simulink model "Stinger"  (R2023a)
settings: Solver=VariableStepAuto  StartTime=0.0  StopTime=20  FixedStep=1e-3  EnableMultiTasking=on
values from neighbouring files (symbols this model uses):
  bp = 0.001    [ControlLawsScript.m]    (also in ControlLaws_Script.m)
  bq = 0.001    [ControlLawsScript.m]    (also in ControlLaws_Script.m)
  br = 0.001    [ControlLawsScript.m]    (also in ControlLaws_Script.m)
  cx = 5    [ControlLawsScript.m]    (also in ControlLaws_Script.m)
  cy = 5    [ControlLawsScript.m]    (also in ControlLaws_Script.m)
  cz = 5    [ControlLawsScript.m]    (also in ControlLaws_Script.m)
  g = 9.80665    [ControlLawsScript.m]    (also in ControlLaws_Script.m; Qball_X8_Model.m = 9.87)
  Kp = (Jx/Tc)-bp    (= 1.02772632451)    [ControlLawsScript.m]    (also in ControlLaws_Script.m = 4.11390529802)
  Kp2 = Jx*((4/ts))*((-4/ts)+((bp+Kp)/Jx))/Kp    (= 1.68163467643)    [ControlLawsScript.m]    (also in ControlLaws_Script.m = 6.72163348437)
  Kq = (Jy/Tc)-bq    (= 1.02971502036)    [ControlLawsScript.m]    (also in ControlLaws_Script.m = 4.12186008142)
  Kq2 = Jy*((4/ts))*((-4/ts)+((bq+Kq)/Jy))/Kq    (= 1.68163151937)    [ControlLawsScript.m]    (also in ControlLaws_Script.m = 6.72163033191)
  Kr = (Jz/Tc)-br    (= 1.98490876719)    [ControlLawsScript.m]    (also in ControlLaws_Script.m = 7.94263506876)
  Kr2 = Jz*((4/ts))*((-4/ts)+((br+Kr)/Jz))/Kr    (= 1.68084638651)    [ControlLawsScript.m]    (also in ControlLaws_Script.m = 6.72084606682)
  kv = 1/930    (= 0.0010752688172)    [StingerScript.m]
  Kx = abs(Kx)    [ControlLawsScript.m]    (also in ControlLaws_Script.m)
  Ky = abs(Ky)    [ControlLawsScript.m]    (also in ControlLaws_Script.m)
  Kz = (m/Tcz)-cz    (= 38.5143536865)    [ControlLawsScript.m]    (also in ControlLaws_Script.m)
  Kz2 = m*((4/tsz))*((-4/tsz)+((cz+Kz)/m))/Kz    (= 1.89810050529)    [ControlLawsScript.m]    (also in ControlLaws_Script.m)
  m = 3.4811482949175    (= 3.48114829492)    [ControlLawsScript.m]    (also in ControlLaws_Script.m; Qball_X8_Model.m = 1.45)
  pitch_angle_limit = pi/6    (= 0.523598775598)    [ControlLawsScript.m]    (also in ControlLaws_Script.m = 0.558505360638)
  R2D = 180/pi    (= 57.2957795131)    [ControlLawsScript.m]    (also in ControlLaws_Script.m)
  roll_angle_limit = pi/6    (= 0.523598775598)    [ControlLawsScript.m]    (also in ControlLaws_Script.m = 0.558505360638)
  z_x = cx    (= 5)    [ControlLawsScript.m]    (also in ControlLaws_Script.m)
  z_y = cy    (= 5)    [ControlLawsScript.m]    (also in ControlLaws_Script.m)
undefined symbols (not defined in the file or in its folder): FC, LAC, LeftAftArm, LeftAftProp, LeftAftSkid, LeftArm, LeftFrontArm, LeftFrontProp, LeftFrontSkid, LeftProp, Lower, missionPlanX, missionPlanY, missionPlanYaw, missionPlanZ, RAC, RightAftArm, RightAftProp, RightAftSkid, RightArm, RightFrontArm, RightFrontProp, RightFrontSkid, RightProp, SC, timeConstant, Upper, X, Y, Z
libraries: sm_lib x98, nesl_utility x56, fl_lib x45, ee_lib x19, batteryecm_lib x2, sharedtransformsys x1, sharedutil x1
(part 3 of 4)

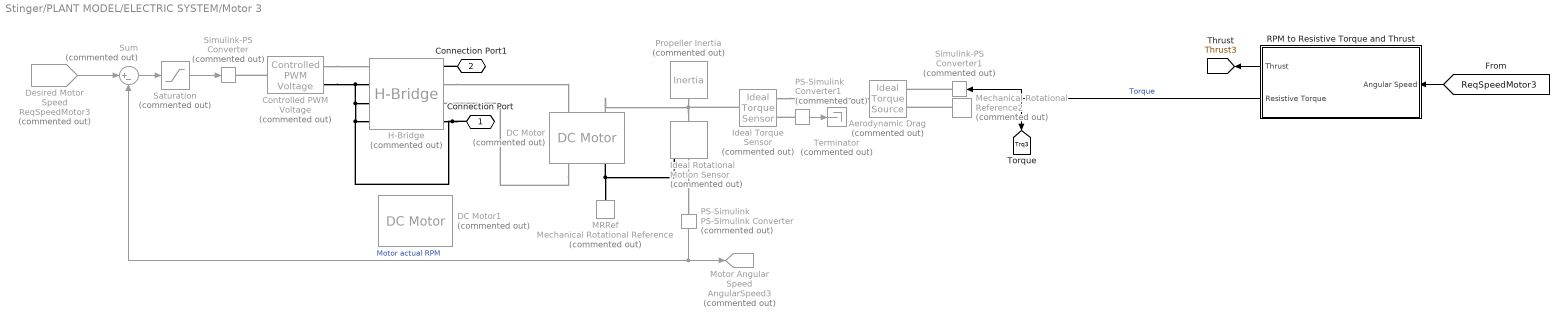
== system Stinger/PLANT MODEL/ELECTRIC SYSTEM/Motor 3 ==
  Aerodynamic Drag : fl_lib/Mechanical/Mechanical Sources/Ideal Torque Source  Commented=on
  Controlled PWM Voltage : ee_lib/Integrated Circuits/Controlled PWM Voltage  Commented=on  F=200 Hz  TD=0 s  pulse_width_offset=0 s  pulse_min=0 s  pwm_or_av=1  event_type=1  sample_time=5e-6 s  Vmin=0 V  Vmax=5 V  Vm=1 V  u_min=0  u_max=1
      settings: InternalSimscapePortConfiguration="{\"Bottom\":[],\"Left\":[{\"id\":\"u\",\"label\":\"u\",\"type\":\"input\"}],\"Right\":[{\"id\":\"p2\",\"label\":\"PWM\",\"type\":\"foundation.electrical.electrical\"},{\"id\":\"n2\",\"label\":\"REF\",\"type\":\"foundation.electrical.electrical\"}],\"Top\":[]}"
  DC Motor : ee_lib/Electromechanical/Brushed Motors/DC Motor  Commented=on  field_option=ee.enum.field_option.pm  Rf=100 Ohm  Lf=1 H  Laf=0.15 H  If0=0 A  parameterization=ee.enum.dcparam_option.circuit_param  Ra=R Ohm  La=100 uH  emf_or_torque=ee.enum.emf_or_torque.kv  Kv=kv V/rpm  Ki=kv N*m/A  T_stall=0.1 N*m  w_max=4000 rpm  w_rated=2500 rpm  P_rated=10 W  V_rated=12 V  lam_param=ee.enum.lam_param.current  i_noload=Ic A  V_i_noload=14.8 V  J=0 kg*m^2  lam=0.5e-5 N*m/(rad/s)  speed0=0 rpm  enable_fault_armature=simscape.enum.onoff.off  rev_faulted=1 / 3  G_faulted_armature=1e-5 S  fault_trigger_armature=ee.enum.faults.faultTrigger.temporal  t_fault_armature=1 s  max_permissible_current_armature=inf A  t_fail_on_current_armature=1 s  enable_fault_field=simscape.enum.onoff.off  G_faulted_field=1e-5 S  fault_trigger_field=ee.enum.faults.faultTrigger.temporal  t_fault_field=1 s  max_permissible_current_field=inf A  t_fail_on_current_field=1 s  fault_action=simscape.enum.assert.action.none  alpha=3.93e-3 1/K  Tmeas=25 degC  thermal_mass=100 J/K  initial_temperature=25 degC
  DC Motor1 : ee_lib/Electromechanical/Brushed Motors/DC Motor  Commented=on  field_option=ee.enum.field_option.pm  Rf=100 Ohm  Lf=1 H  Laf=0.15 H  If0=0 A  parameterization=ee.enum.dcparam_option.circuit_param  Ra=R Ohm  La=100 uH  emf_or_torque=ee.enum.emf_or_torque.kv  Kv=kv V/rpm  Ki=kv N*m/A  T_stall=0.1 N*m  w_max=4000 rpm  w_rated=2500 rpm  P_rated=10 W  V_rated=12 V  lam_param=ee.enum.lam_param.current  i_noload=Ic A  V_i_noload=14.8 V  J=0 kg*m^2  lam=0.5e-5 N*m/(rad/s)  speed0=0 rpm  enable_fault_armature=simscape.enum.onoff.off  rev_faulted=1 / 3  G_faulted_armature=1e-5 S  fault_trigger_armature=ee.enum.faults.faultTrigger.temporal  t_fault_armature=1 s  max_permissible_current_armature=inf A  t_fail_on_current_armature=1 s  enable_fault_field=simscape.enum.onoff.off  G_faulted_field=1e-5 S  fault_trigger_field=ee.enum.faults.faultTrigger.temporal  t_fault_field=1 s  max_permissible_current_field=inf A  t_fail_on_current_field=1 s  fault_action=simscape.enum.assert.action.none  alpha=3.93e-3 1/K  Tmeas=25 degC  thermal_mass=100 J/K  initial_temperature=25 degC
  Desired Motor Speed : From  Commented=on  GotoTag=ReqSpeedMotor3  TagVisibility=global
  H-Bridge : ee_lib/Semiconductors & Converters/Converters/H-Bridge  Commented=on  supply_ports=ee.enum.supply_ports.showsupply  pwm_or_av=ee.enum.pwm_or_av.pwm  regenerative_braking_mode=ee.enum.converters.regenerative_braking_mode.always_enabled  discontinuous=ee.enum.current_profile.continuous  freewheeling_mode=ee.enum.converters.freewheeling_mode.two_switches_one_diode  Rload=3.38+0.1 Ohm  Lload=1e-5 H  F=4 kHz  Venable=0.01 V  Vmax=5 V  Vreverse=10000 V  Vbrake=10000 V  Vm=12 V  Ron=0.00001 Ohm  Don=0.1 Ohm  Goff=1e-6 S  Tmeas=298.15 K  Ron2=0.1 Ohm  Don2=0.05 Ohm  Tmeas2=398.15 K  thermal_mass=100 J/K  initial_temperature=298.15 K
      settings: InternalSimscapePortConfiguration="{\"Bottom\":[],\"Left\":[{\"id\":\"ENA\",\"label\":\"PWM\",\"type\":\"foundation.electrical.electrical\"},{\"id\":\"REF\",\"label\":\"REF\",\"type\":\"foundation.electrical.electrical\"},{\"id\":\"REV\",\"label\":\"REV\",\"type\":\"foundation.electrical.electrical\"},{\"id\":\"BRK\",\"label\":\"BRK\",\"type\":\"foundation.electrical.electrical\"}],\"Right\":[{\"id\":\"p1\",\"label\":\"V+\",\"type\":\"foundation.electrical.electrical\"},{\"id\":\"p2\",\"label\":\"+\",\"type\":\"foundation.electrical.electrical\"},{\"id\":\"n2\",\"label\":\"-\",\"type\":\"foundation.electrical.electrical\"},{\"id\":\"n1\",\"label\":\"V-\",\"type\":\"foundation.electrical.electrical\"}],\"Top\":[]}"
  Ideal Rotational Motion Sensor : fl_lib/Mechanical/Mechanical Sensors/Ideal Rotational Motion Sensor  Commented=on  reference=foundation.enum.MeasurementReference.difference  acceleration_port=false  velocity_port=true  position_port=true  wrap_angle=simscape.enum.onoff.off  offset=0 deg
  Ideal Torque Sensor : fl_lib/Mechanical/Mechanical Sensors/Ideal Torque Sensor  Commented=on
  MRRef : fl_lib/Mechanical/Rotational Elements/Mechanical Rotational Reference  Commented=on
  Mechanical Rotational Reference2 : fl_lib/Mechanical/Rotational Elements/Mechanical Rotational Reference  Commented=on
  Motor Angular Speed : Goto  Commented=on  GotoTag=AngularSpeed3  TagVisibility=global
  PS-Simulink : nesl_utility/PS-Simulink Converter  Commented=on  PhysicalDomain=network_engine_domain  SubClassName=ps_output  LeftPortType=input  RightPortType=output  PseudoPeriodic=off  Frequencies=[]  VectorFormat=1-D array  Unit=rpm  AffineConversion=off
  PS-Simulink Converter1 : nesl_utility/PS-Simulink Converter  Commented=on  PhysicalDomain=network_engine_domain  SubClassName=ps_output  LeftPortType=input  RightPortType=output  PseudoPeriodic=off  Frequencies=[]  VectorFormat=1-D array  Unit=inherit  AffineConversion=off
  Propeller Inertia : fl_lib/Mechanical/Rotational Elements/Inertia  Commented=on  inertia=J kg*m^2  num_ports=foundation.enum.numPorts2.one  w_specify=off  w_priority=High  w=0 rpm  w_nominal_specify=off  w_nominal_unit=rad/s  w_nominal_value=1  t_specify=off  t_priority=High  t=0 N*m  t_nominal_specify=off  t_nominal_unit=N*m  t_nominal_value=1
  RPM to Resistive Torque and Thrust : Subsystem
  Saturation : Saturate  Commented=on  UpperLimit=1  LowerLimit=0
  Simulink-PS Converter : nesl_utility/Simulink-PS Converter  Commented=on  PhysicalDomain=network_engine_domain  SubClassName=ps_input  LeftPortType=input  RightPortType=output  PseudoPeriodic=off  Frequencies=[]  NoiseDistribution=none  NoiseParameters=[]  Unit=1  AffineConversion=off  FilteringAndDerivatives=provide  SimscapeFilterOrder=1  InputFilterTimeConstant=0.001  UdotUserProvided=0
  Simulink-PS Converter1 : nesl_utility/Simulink-PS Converter  Commented=on  PhysicalDomain=network_engine_domain  SubClassName=ps_input  LeftPortType=input  RightPortType=output  PseudoPeriodic=off  Frequencies=[]  NoiseDistribution=none  NoiseParameters=[]  Unit=N*m  AffineConversion=off  FilteringAndDerivatives=provide  SimscapeFilterOrder=1  InputFilterTimeConstant=0.001  UdotUserProvided=0
  Sum : Sum  Commented=on  Inputs=|+-
  Terminator : Terminator  Commented=on
  Connection Port : PMIOPort  Side=Left
  Connection Port1 : PMIOPort  Port=2  Side=Right
  tag scope: Thrust3=global, Trq3=global
  wires:
  RPM to Resistive Torque and Thrust/2(Resistive Torque) -> Simulink-PS Converter1/1, [Trq3]  "Torque"
  [ReqSpeedMotor3] -> RPM to Resistive Torque and Thrust/1(Angular Speed)
  RPM to Resistive Torque and Thrust/1(Thrust) -> [Thrust3]
  PS-Simulink Converter1/1 -> Terminator/1
  PS-Simulink/1 -> Sum/2, Motor Angular Speed/1  "Motor actual RPM"
  Desired Motor Speed/1 -> Sum/1
  Sum/1 -> Saturation/1
  Saturation/1 -> Simulink-PS Converter/1
  connections:
  Ideal Rotational Motion Sensor/RConn2 -- PS-Simulink/LConn1
  PS-Simulink Converter1/LConn1 -- Ideal Torque Sensor/RConn2
  Ideal Torque Sensor/RConn1 -- Aerodynamic Drag/LConn1
  Simulink-PS Converter1/RConn1 -- Aerodynamic Drag/RConn1
  Mechanical Rotational Reference2/LConn1 -- Aerodynamic Drag/RConn2
  Ideal Torque Sensor/LConn1 -- DC Motor/LConn2 -- Propeller Inertia/LConn1 -- Ideal Rotational Motion Sensor/LConn1
  Ideal Rotational Motion Sensor/RConn1 -- MRRef/LConn1 -- DC Motor/RConn2
  H-Bridge/LConn4 -- H-Bridge/RConn4 -- Connection Port/RConn1 -- H-Bridge/LConn3 -- Controlled PWM Voltage/RConn2 -- H-Bridge/LConn2
  H-Bridge/RConn2 -- DC Motor/LConn1
  Controlled PWM Voltage/RConn1 -- H-Bridge/LConn1
  Controlled PWM Voltage/LConn1 -- Simulink-PS Converter/RConn1
  DC Motor/RConn1 -- H-Bridge/RConn3
  Connection Port1/RConn1 -- H-Bridge/RConn1

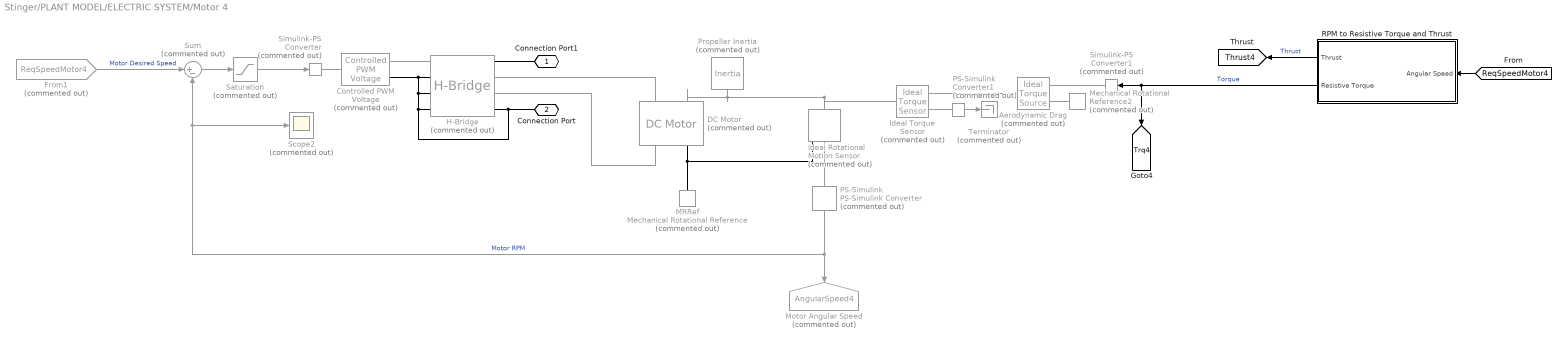
== system Stinger/PLANT MODEL/ELECTRIC SYSTEM/Motor 4 ==
  Aerodynamic Drag : fl_lib/Mechanical/Mechanical Sources/Ideal Torque Source  Commented=on
  Controlled PWM Voltage : ee_lib/Integrated Circuits/Controlled PWM Voltage  Commented=on  F=200 Hz  TD=0 s  pulse_width_offset=0 s  pulse_min=0 s  pwm_or_av=1  event_type=1  sample_time=5e-6 s  Vmin=0 V  Vmax=5 V  Vm=1 V  u_min=0  u_max=1
      settings: InternalSimscapePortConfiguration="{\"Bottom\":[],\"Left\":[{\"id\":\"u\",\"label\":\"u\",\"type\":\"input\"}],\"Right\":[{\"id\":\"p2\",\"label\":\"PWM\",\"type\":\"foundation.electrical.electrical\"},{\"id\":\"n2\",\"label\":\"REF\",\"type\":\"foundation.electrical.electrical\"}],\"Top\":[]}"
  DC Motor : ee_lib/Electromechanical/Brushed Motors/DC Motor  Commented=on  field_option=ee.enum.field_option.pm  Rf=100 Ohm  Lf=1 H  Laf=0.15 H  If0=0 A  parameterization=ee.enum.dcparam_option.circuit_param  Ra=R Ohm  La=100 uH  emf_or_torque=ee.enum.emf_or_torque.kv  Kv=kv V/rpm  Ki=kv N*m/A  T_stall=0.1 N*m  w_max=4000 rpm  w_rated=2500 rpm  P_rated=10 W  V_rated=12 V  lam_param=ee.enum.lam_param.current  i_noload=Ic A  V_i_noload=14.8 V  J=0 kg*m^2  lam=0.5e-5 N*m/(rad/s)  speed0=0 rpm  enable_fault_armature=simscape.enum.onoff.off  rev_faulted=1 / 3  G_faulted_armature=1e-5 S  fault_trigger_armature=ee.enum.faults.faultTrigger.temporal  t_fault_armature=1 s  max_permissible_current_armature=inf A  t_fail_on_current_armature=1 s  enable_fault_field=simscape.enum.onoff.off  G_faulted_field=1e-5 S  fault_trigger_field=ee.enum.faults.faultTrigger.temporal  t_fault_field=1 s  max_permissible_current_field=inf A  t_fail_on_current_field=1 s  fault_action=simscape.enum.assert.action.none  alpha=3.93e-3 1/K  Tmeas=25 degC  thermal_mass=100 J/K  initial_temperature=25 degC
  From1 : From  Commented=on  GotoTag=ReqSpeedMotor4  TagVisibility=global
  H-Bridge : ee_lib/Semiconductors & Converters/Converters/H-Bridge  Commented=on  supply_ports=ee.enum.supply_ports.showsupply  pwm_or_av=ee.enum.pwm_or_av.pwm  regenerative_braking_mode=ee.enum.converters.regenerative_braking_mode.always_enabled  discontinuous=ee.enum.current_profile.continuous  freewheeling_mode=ee.enum.converters.freewheeling_mode.two_switches_one_diode  Rload=3.38+0.1 Ohm  Lload=1e-5 H  F=4 kHz  Venable=0.01 V  Vmax=5 V  Vreverse=10000 V  Vbrake=10000 V  Vm=12 V  Ron=0.00001 Ohm  Don=0.1 Ohm  Goff=1e-6 S  Tmeas=298.15 K  Ron2=0.1 Ohm  Don2=0.05 Ohm  Tmeas2=398.15 K  thermal_mass=100 J/K  initial_temperature=298.15 K
      settings: InternalSimscapePortConfiguration="{\"Bottom\":[],\"Left\":[{\"id\":\"ENA\",\"label\":\"PWM\",\"type\":\"foundation.electrical.electrical\"},{\"id\":\"REF\",\"label\":\"REF\",\"type\":\"foundation.electrical.electrical\"},{\"id\":\"REV\",\"label\":\"REV\",\"type\":\"foundation.electrical.electrical\"},{\"id\":\"BRK\",\"label\":\"BRK\",\"type\":\"foundation.electrical.electrical\"}],\"Right\":[{\"id\":\"p1\",\"label\":\"V+\",\"type\":\"foundation.electrical.electrical\"},{\"id\":\"p2\",\"label\":\"+\",\"type\":\"foundation.electrical.electrical\"},{\"id\":\"n2\",\"label\":\"-\",\"type\":\"foundation.electrical.electrical\"},{\"id\":\"n1\",\"label\":\"V-\",\"type\":\"foundation.electrical.electrical\"}],\"Top\":[]}"
  Ideal Rotational Motion Sensor : fl_lib/Mechanical/Mechanical Sensors/Ideal Rotational Motion Sensor  Commented=on  reference=foundation.enum.MeasurementReference.difference  acceleration_port=false  velocity_port=true  position_port=true  wrap_angle=simscape.enum.onoff.off  offset=0 deg
  Ideal Torque Sensor : fl_lib/Mechanical/Mechanical Sensors/Ideal Torque Sensor  Commented=on
  MRRef : fl_lib/Mechanical/Rotational Elements/Mechanical Rotational Reference  Commented=on
  Mechanical Rotational Reference2 : fl_lib/Mechanical/Rotational Elements/Mechanical Rotational Reference  Commented=on
  Motor Angular Speed : Goto  Commented=on  GotoTag=AngularSpeed4  TagVisibility=global
  PS-Simulink : nesl_utility/PS-Simulink Converter  Commented=on  PhysicalDomain=network_engine_domain  SubClassName=ps_output  LeftPortType=input  RightPortType=output  PseudoPeriodic=off  Frequencies=[]  VectorFormat=1-D array  Unit=rpm  AffineConversion=off
  PS-Simulink Converter1 : nesl_utility/PS-Simulink Converter  Commented=on  PhysicalDomain=network_engine_domain  SubClassName=ps_output  LeftPortType=input  RightPortType=output  PseudoPeriodic=off  Frequencies=[]  VectorFormat=1-D array  Unit=inherit  AffineConversion=off
  Propeller Inertia : fl_lib/Mechanical/Rotational Elements/Inertia  Commented=on  inertia=J kg*m^2  num_ports=foundation.enum.numPorts2.one  w_specify=off  w_priority=High  w=0 rpm  w_nominal_specify=off  w_nominal_unit=rad/s  w_nominal_value=1  t_specify=off  t_priority=High  t=0 N*m  t_nominal_specify=off  t_nominal_unit=N*m  t_nominal_value=1
  RPM to Resistive Torque and Thrust : Subsystem
  Saturation : Saturate  Commented=on  UpperLimit=1  LowerLimit=0
  Scope2 : Scope  Commented=on
  Simulink-PS Converter : nesl_utility/Simulink-PS Converter  Commented=on  PhysicalDomain=network_engine_domain  SubClassName=ps_input  LeftPortType=input  RightPortType=output  PseudoPeriodic=off  Frequencies=[]  NoiseDistribution=none  NoiseParameters=[]  Unit=1  AffineConversion=off  FilteringAndDerivatives=provide  SimscapeFilterOrder=1  InputFilterTimeConstant=0.001  UdotUserProvided=0
  Simulink-PS Converter1 : nesl_utility/Simulink-PS Converter  Commented=on  PhysicalDomain=network_engine_domain  SubClassName=ps_input  LeftPortType=input  RightPortType=output  PseudoPeriodic=off  Frequencies=[]  NoiseDistribution=none  NoiseParameters=[]  Unit=N*m  AffineConversion=off  FilteringAndDerivatives=provide  SimscapeFilterOrder=1  InputFilterTimeConstant=0.001  UdotUserProvided=0
  Sum : Sum  Commented=on  Inputs=|+-
  Terminator : Terminator  Commented=on
  Connection Port1 : PMIOPort  Side=Left
  Connection Port : PMIOPort  Port=2  Side=Right
  tag scope: Thrust4=global, Trq4=global
  wires:
  RPM to Resistive Torque and Thrust/2(Resistive Torque) -> [Trq4], Simulink-PS Converter1/1  "Torque"
  [ReqSpeedMotor4] -> RPM to Resistive Torque and Thrust/1(Angular Speed)
  RPM to Resistive Torque and Thrust/1(Thrust) -> [Thrust4]  "Thrust"
  PS-Simulink Converter1/1 -> Terminator/1
  PS-Simulink/1 -> Scope2/1, Sum/2, Motor Angular Speed/1  "Motor RPM"
  From1/1 -> Sum/1  "Motor Desired Speed"
  Sum/1 -> Saturation/1
  Saturation/1 -> Simulink-PS Converter/1
  connections:
  Ideal Rotational Motion Sensor/RConn2 -- PS-Simulink/LConn1
  PS-Simulink Converter1/LConn1 -- Ideal Torque Sensor/RConn2
  Ideal Torque Sensor/RConn1 -- Aerodynamic Drag/LConn1
  Simulink-PS Converter1/RConn1 -- Aerodynamic Drag/RConn1
  Mechanical Rotational Reference2/LConn1 -- Aerodynamic Drag/RConn2
  Ideal Torque Sensor/LConn1 -- DC Motor/LConn2 -- Propeller Inertia/LConn1 -- Ideal Rotational Motion Sensor/LConn1
  Ideal Rotational Motion Sensor/RConn1 -- MRRef/LConn1 -- DC Motor/RConn2
  H-Bridge/RConn4 -- Connection Port/RConn1 -- H-Bridge/LConn3 -- Controlled PWM Voltage/RConn2 -- H-Bridge/LConn2 -- H-Bridge/LConn4
  H-Bridge/RConn2 -- DC Motor/LConn1
  Controlled PWM Voltage/RConn1 -- H-Bridge/LConn1
  Controlled PWM Voltage/LConn1 -- Simulink-PS Converter/RConn1
  H-Bridge/RConn3 -- DC Motor/RConn1
  Connection Port1/RConn1 -- H-Bridge/RConn1

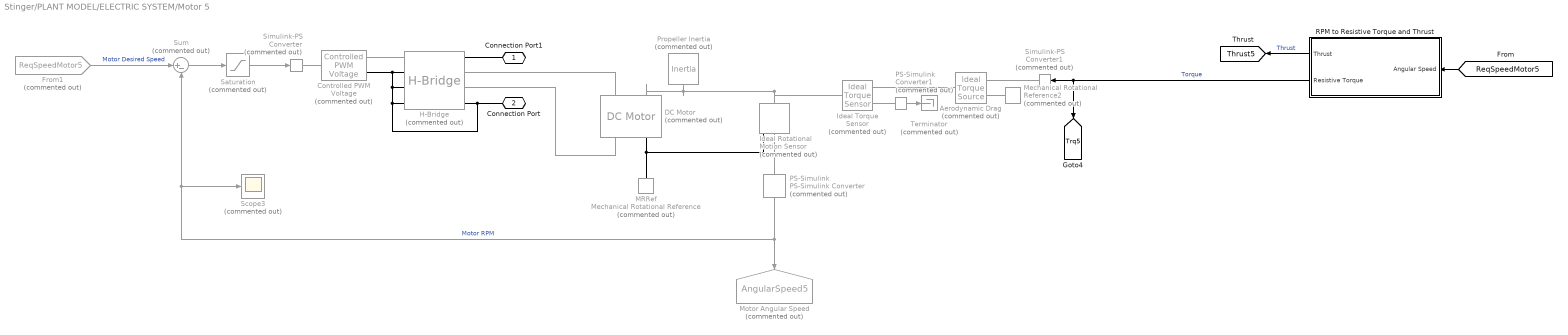
== system Stinger/PLANT MODEL/ELECTRIC SYSTEM/Motor 5 ==
  Aerodynamic Drag : fl_lib/Mechanical/Mechanical Sources/Ideal Torque Source  Commented=on
  Controlled PWM Voltage : ee_lib/Integrated Circuits/Controlled PWM Voltage  Commented=on  F=200 Hz  TD=0 s  pulse_width_offset=0 s  pulse_min=0 s  pwm_or_av=1  event_type=1  sample_time=5e-6 s  Vmin=0 V  Vmax=5 V  Vm=1 V  u_min=0  u_max=1
      settings: InternalSimscapePortConfiguration="{\"Bottom\":[],\"Left\":[{\"id\":\"u\",\"label\":\"u\",\"type\":\"input\"}],\"Right\":[{\"id\":\"p2\",\"label\":\"PWM\",\"type\":\"foundation.electrical.electrical\"},{\"id\":\"n2\",\"label\":\"REF\",\"type\":\"foundation.electrical.electrical\"}],\"Top\":[]}"
  DC Motor : ee_lib/Electromechanical/Brushed Motors/DC Motor  Commented=on  field_option=ee.enum.field_option.pm  Rf=100 Ohm  Lf=1 H  Laf=0.15 H  If0=0 A  parameterization=ee.enum.dcparam_option.circuit_param  Ra=R Ohm  La=100 uH  emf_or_torque=ee.enum.emf_or_torque.kv  Kv=kv V/rpm  Ki=kv N*m/A  T_stall=0.1 N*m  w_max=4000 rpm  w_rated=2500 rpm  P_rated=10 W  V_rated=12 V  lam_param=ee.enum.lam_param.current  i_noload=Ic A  V_i_noload=14.8 V  J=0 kg*m^2  lam=0.5e-5 N*m/(rad/s)  speed0=0 rpm  enable_fault_armature=simscape.enum.onoff.off  rev_faulted=1 / 3  G_faulted_armature=1e-5 S  fault_trigger_armature=ee.enum.faults.faultTrigger.temporal  t_fault_armature=1 s  max_permissible_current_armature=inf A  t_fail_on_current_armature=1 s  enable_fault_field=simscape.enum.onoff.off  G_faulted_field=1e-5 S  fault_trigger_field=ee.enum.faults.faultTrigger.temporal  t_fault_field=1 s  max_permissible_current_field=inf A  t_fail_on_current_field=1 s  fault_action=simscape.enum.assert.action.none  alpha=3.93e-3 1/K  Tmeas=25 degC  thermal_mass=100 J/K  initial_temperature=25 degC
  From1 : From  Commented=on  GotoTag=ReqSpeedMotor5  TagVisibility=global
  H-Bridge : ee_lib/Semiconductors & Converters/Converters/H-Bridge  Commented=on  supply_ports=ee.enum.supply_ports.showsupply  pwm_or_av=ee.enum.pwm_or_av.pwm  regenerative_braking_mode=ee.enum.converters.regenerative_braking_mode.always_enabled  discontinuous=ee.enum.current_profile.continuous  freewheeling_mode=ee.enum.converters.freewheeling_mode.two_switches_one_diode  Rload=3.38+0.1 Ohm  Lload=1e-5 H  F=4 kHz  Venable=0.01 V  Vmax=5 V  Vreverse=10000 V  Vbrake=10000 V  Vm=12 V  Ron=0.00001 Ohm  Don=0.1 Ohm  Goff=1e-6 S  Tmeas=298.15 K  Ron2=0.1 Ohm  Don2=0.05 Ohm  Tmeas2=398.15 K  thermal_mass=100 J/K  initial_temperature=298.15 K
      settings: InternalSimscapePortConfiguration="{\"Bottom\":[],\"Left\":[{\"id\":\"ENA\",\"label\":\"PWM\",\"type\":\"foundation.electrical.electrical\"},{\"id\":\"REF\",\"label\":\"REF\",\"type\":\"foundation.electrical.electrical\"},{\"id\":\"REV\",\"label\":\"REV\",\"type\":\"foundation.electrical.electrical\"},{\"id\":\"BRK\",\"label\":\"BRK\",\"type\":\"foundation.electrical.electrical\"}],\"Right\":[{\"id\":\"p1\",\"label\":\"V+\",\"type\":\"foundation.electrical.electrical\"},{\"id\":\"p2\",\"label\":\"+\",\"type\":\"foundation.electrical.electrical\"},{\"id\":\"n2\",\"label\":\"-\",\"type\":\"foundation.electrical.electrical\"},{\"id\":\"n1\",\"label\":\"V-\",\"type\":\"foundation.electrical.electrical\"}],\"Top\":[]}"
  Ideal Rotational Motion Sensor : fl_lib/Mechanical/Mechanical Sensors/Ideal Rotational Motion Sensor  Commented=on  reference=foundation.enum.MeasurementReference.difference  acceleration_port=false  velocity_port=true  position_port=true  wrap_angle=simscape.enum.onoff.off  offset=0 deg
  Ideal Torque Sensor : fl_lib/Mechanical/Mechanical Sensors/Ideal Torque Sensor  Commented=on
  MRRef : fl_lib/Mechanical/Rotational Elements/Mechanical Rotational Reference  Commented=on
  Mechanical Rotational Reference2 : fl_lib/Mechanical/Rotational Elements/Mechanical Rotational Reference  Commented=on
  Motor Angular Speed : Goto  Commented=on  GotoTag=AngularSpeed5  TagVisibility=global
  PS-Simulink : nesl_utility/PS-Simulink Converter  Commented=on  PhysicalDomain=network_engine_domain  SubClassName=ps_output  LeftPortType=input  RightPortType=output  PseudoPeriodic=off  Frequencies=[]  VectorFormat=1-D array  Unit=rpm  AffineConversion=off
  PS-Simulink Converter1 : nesl_utility/PS-Simulink Converter  Commented=on  PhysicalDomain=network_engine_domain  SubClassName=ps_output  LeftPortType=input  RightPortType=output  PseudoPeriodic=off  Frequencies=[]  VectorFormat=1-D array  Unit=inherit  AffineConversion=off
  Propeller Inertia : fl_lib/Mechanical/Rotational Elements/Inertia  Commented=on  inertia=J kg*m^2  num_ports=foundation.enum.numPorts2.one  w_specify=off  w_priority=High  w=0 rpm  w_nominal_specify=off  w_nominal_unit=rad/s  w_nominal_value=1  t_specify=off  t_priority=High  t=0 N*m  t_nominal_specify=off  t_nominal_unit=N*m  t_nominal_value=1
  RPM to Resistive Torque and Thrust : Subsystem
  Saturation : Saturate  Commented=on  UpperLimit=1  LowerLimit=0
  Scope3 : Scope  Commented=on
  Simulink-PS Converter : nesl_utility/Simulink-PS Converter  Commented=on  PhysicalDomain=network_engine_domain  SubClassName=ps_input  LeftPortType=input  RightPortType=output  PseudoPeriodic=off  Frequencies=[]  NoiseDistribution=none  NoiseParameters=[]  Unit=1  AffineConversion=off  FilteringAndDerivatives=provide  SimscapeFilterOrder=1  InputFilterTimeConstant=0.001  UdotUserProvided=0
  Simulink-PS Converter1 : nesl_utility/Simulink-PS Converter  Commented=on  PhysicalDomain=network_engine_domain  SubClassName=ps_input  LeftPortType=input  RightPortType=output  PseudoPeriodic=off  Frequencies=[]  NoiseDistribution=none  NoiseParameters=[]  Unit=N*m  AffineConversion=off  FilteringAndDerivatives=provide  SimscapeFilterOrder=1  InputFilterTimeConstant=0.001  UdotUserProvided=0
  Sum : Sum  Commented=on  Inputs=|+-
  Terminator : Terminator  Commented=on
  Connection Port1 : PMIOPort  Side=Left
  Connection Port : PMIOPort  Port=2  Side=Right
  tag scope: Thrust5=global, Trq5=global
  wires:
  RPM to Resistive Torque and Thrust/2(Resistive Torque) -> [Trq5], Simulink-PS Converter1/1  "Torque"
  [ReqSpeedMotor5] -> RPM to Resistive Torque and Thrust/1(Angular Speed)
  RPM to Resistive Torque and Thrust/1(Thrust) -> [Thrust5]  "Thrust"
  PS-Simulink Converter1/1 -> Terminator/1
  PS-Simulink/1 -> Scope3/1, Sum/2, Motor Angular Speed/1  "Motor RPM"
  From1/1 -> Sum/1  "Motor Desired Speed"
  Sum/1 -> Saturation/1
  Saturation/1 -> Simulink-PS Converter/1
  connections:
  Ideal Rotational Motion Sensor/RConn2 -- PS-Simulink/LConn1
  PS-Simulink Converter1/LConn1 -- Ideal Torque Sensor/RConn2
  Ideal Torque Sensor/RConn1 -- Aerodynamic Drag/LConn1
  Simulink-PS Converter1/RConn1 -- Aerodynamic Drag/RConn1
  Mechanical Rotational Reference2/LConn1 -- Aerodynamic Drag/RConn2
  Ideal Torque Sensor/LConn1 -- DC Motor/LConn2 -- Propeller Inertia/LConn1 -- Ideal Rotational Motion Sensor/LConn1
  Ideal Rotational Motion Sensor/RConn1 -- MRRef/LConn1 -- DC Motor/RConn2
  Connection Port/RConn1 -- H-Bridge/RConn4 -- H-Bridge/LConn3 -- Controlled PWM Voltage/RConn2 -- H-Bridge/LConn2 -- H-Bridge/LConn4
  H-Bridge/RConn2 -- DC Motor/LConn1
  Controlled PWM Voltage/RConn1 -- H-Bridge/LConn1
  Controlled PWM Voltage/LConn1 -- Simulink-PS Converter/RConn1
  H-Bridge/RConn3 -- DC Motor/RConn1
  Connection Port1/RConn1 -- H-Bridge/RConn1

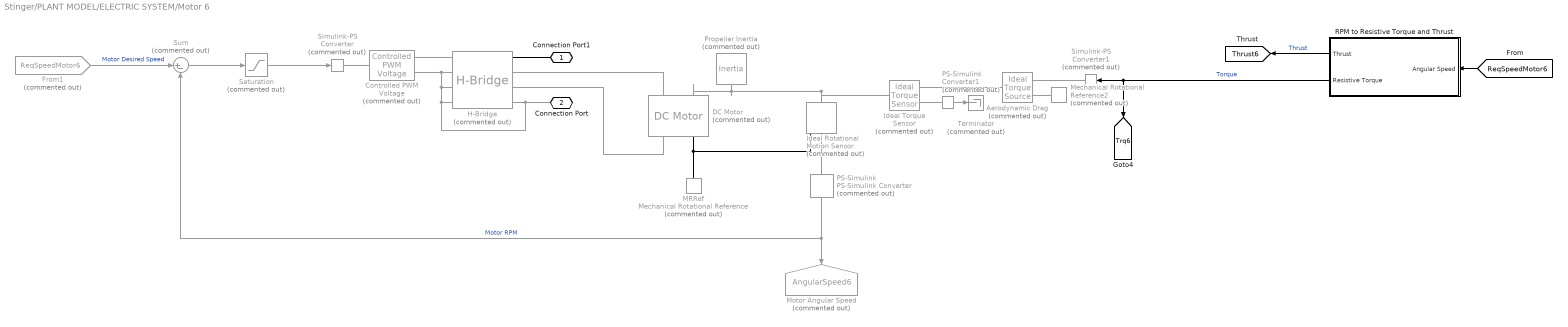
== system Stinger/PLANT MODEL/ELECTRIC SYSTEM/Motor 6 ==
  Aerodynamic Drag : fl_lib/Mechanical/Mechanical Sources/Ideal Torque Source  Commented=on
  Controlled PWM Voltage : ee_lib/Integrated Circuits/Controlled PWM Voltage  Commented=on  F=200 Hz  TD=0 s  pulse_width_offset=0 s  pulse_min=0 s  pwm_or_av=1  event_type=1  sample_time=5e-6 s  Vmin=0 V  Vmax=5 V  Vm=1 V  u_min=0  u_max=1
      settings: InternalSimscapePortConfiguration="{\"Bottom\":[],\"Left\":[{\"id\":\"u\",\"label\":\"u\",\"type\":\"input\"}],\"Right\":[{\"id\":\"p2\",\"label\":\"PWM\",\"type\":\"foundation.electrical.electrical\"},{\"id\":\"n2\",\"label\":\"REF\",\"type\":\"foundation.electrical.electrical\"}],\"Top\":[]}"
  DC Motor : ee_lib/Electromechanical/Brushed Motors/DC Motor  Commented=on  field_option=ee.enum.field_option.pm  Rf=100 Ohm  Lf=1 H  Laf=0.15 H  If0=0 A  parameterization=ee.enum.dcparam_option.circuit_param  Ra=R Ohm  La=100 uH  emf_or_torque=ee.enum.emf_or_torque.kv  Kv=kv V/rpm  Ki=kv N*m/A  T_stall=0.1 N*m  w_max=4000 rpm  w_rated=2500 rpm  P_rated=10 W  V_rated=12 V  lam_param=ee.enum.lam_param.current  i_noload=Ic A  V_i_noload=14.8 V  J=0 kg*m^2  lam=0.5e-5 N*m/(rad/s)  speed0=0 rpm  enable_fault_armature=simscape.enum.onoff.off  rev_faulted=1 / 3  G_faulted_armature=1e-5 S  fault_trigger_armature=ee.enum.faults.faultTrigger.temporal  t_fault_armature=1 s  max_permissible_current_armature=inf A  t_fail_on_current_armature=1 s  enable_fault_field=simscape.enum.onoff.off  G_faulted_field=1e-5 S  fault_trigger_field=ee.enum.faults.faultTrigger.temporal  t_fault_field=1 s  max_permissible_current_field=inf A  t_fail_on_current_field=1 s  fault_action=simscape.enum.assert.action.none  alpha=3.93e-3 1/K  Tmeas=25 degC  thermal_mass=100 J/K  initial_temperature=25 degC
  From1 : From  Commented=on  GotoTag=ReqSpeedMotor6  TagVisibility=global
  H-Bridge : ee_lib/Semiconductors & Converters/Converters/H-Bridge  Commented=on  supply_ports=ee.enum.supply_ports.showsupply  pwm_or_av=ee.enum.pwm_or_av.pwm  regenerative_braking_mode=ee.enum.converters.regenerative_braking_mode.always_enabled  discontinuous=ee.enum.current_profile.continuous  freewheeling_mode=ee.enum.converters.freewheeling_mode.two_switches_one_diode  Rload=3.38+0.1 Ohm  Lload=1e-5 H  F=4 kHz  Venable=0.01 V  Vmax=5 V  Vreverse=10000 V  Vbrake=10000 V  Vm=12 V  Ron=0.00001 Ohm  Don=0.1 Ohm  Goff=1e-6 S  Tmeas=298.15 K  Ron2=0.1 Ohm  Don2=0.05 Ohm  Tmeas2=398.15 K  thermal_mass=100 J/K  initial_temperature=298.15 K
      settings: InternalSimscapePortConfiguration="{\"Bottom\":[],\"Left\":[{\"id\":\"ENA\",\"label\":\"PWM\",\"type\":\"foundation.electrical.electrical\"},{\"id\":\"REF\",\"label\":\"REF\",\"type\":\"foundation.electrical.electrical\"},{\"id\":\"REV\",\"label\":\"REV\",\"type\":\"foundation.electrical.electrical\"},{\"id\":\"BRK\",\"label\":\"BRK\",\"type\":\"foundation.electrical.electrical\"}],\"Right\":[{\"id\":\"p1\",\"label\":\"V+\",\"type\":\"foundation.electrical.electrical\"},{\"id\":\"p2\",\"label\":\"+\",\"type\":\"foundation.electrical.electrical\"},{\"id\":\"n2\",\"label\":\"-\",\"type\":\"foundation.electrical.electrical\"},{\"id\":\"n1\",\"label\":\"V-\",\"type\":\"foundation.electrical.electrical\"}],\"Top\":[]}"
  Ideal Rotational Motion Sensor : fl_lib/Mechanical/Mechanical Sensors/Ideal Rotational Motion Sensor  Commented=on  reference=foundation.enum.MeasurementReference.difference  acceleration_port=false  velocity_port=true  position_port=true  wrap_angle=simscape.enum.onoff.off  offset=0 deg
  Ideal Torque Sensor : fl_lib/Mechanical/Mechanical Sensors/Ideal Torque Sensor  Commented=on
  MRRef : fl_lib/Mechanical/Rotational Elements/Mechanical Rotational Reference  Commented=on
  Mechanical Rotational Reference2 : fl_lib/Mechanical/Rotational Elements/Mechanical Rotational Reference  Commented=on
  Motor Angular Speed : Goto  Commented=on  GotoTag=AngularSpeed6  TagVisibility=global
  PS-Simulink : nesl_utility/PS-Simulink Converter  Commented=on  PhysicalDomain=network_engine_domain  SubClassName=ps_output  LeftPortType=input  RightPortType=output  PseudoPeriodic=off  Frequencies=[]  VectorFormat=1-D array  Unit=rpm  AffineConversion=off
  PS-Simulink Converter1 : nesl_utility/PS-Simulink Converter  Commented=on  PhysicalDomain=network_engine_domain  SubClassName=ps_output  LeftPortType=input  RightPortType=output  PseudoPeriodic=off  Frequencies=[]  VectorFormat=1-D array  Unit=inherit  AffineConversion=off
  Propeller Inertia : fl_lib/Mechanical/Rotational Elements/Inertia  Commented=on  inertia=J kg*m^2  num_ports=foundation.enum.numPorts2.one  w_specify=off  w_priority=High  w=0 rpm  w_nominal_specify=off  w_nominal_unit=rad/s  w_nominal_value=1  t_specify=off  t_priority=High  t=0 N*m  t_nominal_specify=off  t_nominal_unit=N*m  t_nominal_value=1
  RPM to Resistive Torque and Thrust : Subsystem
  Saturation : Saturate  Commented=on  UpperLimit=1  LowerLimit=0
  Simulink-PS Converter : nesl_utility/Simulink-PS Converter  Commented=on  PhysicalDomain=network_engine_domain  SubClassName=ps_input  LeftPortType=input  RightPortType=output  PseudoPeriodic=off  Frequencies=[]  NoiseDistribution=none  NoiseParameters=[]  Unit=1  AffineConversion=off  FilteringAndDerivatives=provide  SimscapeFilterOrder=1  InputFilterTimeConstant=0.001  UdotUserProvided=0
  Simulink-PS Converter1 : nesl_utility/Simulink-PS Converter  Commented=on  PhysicalDomain=network_engine_domain  SubClassName=ps_input  LeftPortType=input  RightPortType=output  PseudoPeriodic=off  Frequencies=[]  NoiseDistribution=none  NoiseParameters=[]  Unit=N*m  AffineConversion=off  FilteringAndDerivatives=provide  SimscapeFilterOrder=1  InputFilterTimeConstant=0.001  UdotUserProvided=0
  Sum : Sum  Commented=on  Inputs=|+-
  Terminator : Terminator  Commented=on
  Connection Port1 : PMIOPort  Side=Left
  Connection Port : PMIOPort  Port=2  Side=Right
  tag scope: Thrust6=global, Trq6=global
  wires:
  RPM to Resistive Torque and Thrust/2(Resistive Torque) -> Simulink-PS Converter1/1, [Trq6]  "Torque"
  [ReqSpeedMotor6] -> RPM to Resistive Torque and Thrust/1(Angular Speed)
  RPM to Resistive Torque and Thrust/1(Thrust) -> [Thrust6]  "Thrust"
  PS-Simulink Converter1/1 -> Terminator/1
  PS-Simulink/1 -> Sum/2, Motor Angular Speed/1  "Motor RPM"
  From1/1 -> Sum/1  "Motor Desired Speed"
  Sum/1 -> Saturation/1
  Saturation/1 -> Simulink-PS Converter/1
  connections:
  Ideal Rotational Motion Sensor/RConn2 -- PS-Simulink/LConn1
  PS-Simulink Converter1/LConn1 -- Ideal Torque Sensor/RConn2
  Ideal Torque Sensor/RConn1 -- Aerodynamic Drag/LConn1
  Simulink-PS Converter1/RConn1 -- Aerodynamic Drag/RConn1
  Mechanical Rotational Reference2/LConn1 -- Aerodynamic Drag/RConn2
  Ideal Torque Sensor/LConn1 -- DC Motor/LConn2 -- Propeller Inertia/LConn1 -- Ideal Rotational Motion Sensor/LConn1
  Ideal Rotational Motion Sensor/RConn1 -- MRRef/LConn1 -- DC Motor/RConn2
  H-Bridge/RConn4 -- H-Bridge/LConn3 -- Controlled PWM Voltage/RConn2 -- H-Bridge/LConn2 -- H-Bridge/LConn4 -- Connection Port/RConn1
  H-Bridge/RConn2 -- DC Motor/LConn1
  Controlled PWM Voltage/RConn1 -- H-Bridge/LConn1
  Controlled PWM Voltage/LConn1 -- Simulink-PS Converter/RConn1
  DC Motor/RConn1 -- H-Bridge/RConn3
  Connection Port1/RConn1 -- H-Bridge/RConn1

== system Stinger/PLANT MODEL/ENVIRONMENT/Ground ==
  Displacement : sm_lib/Frames and Transforms/Rigid Transform  TranslationMethod=StandardAxis  TranslationStandardOffset=P/2+Z+0.01  TranslationStandardOffsetUnits=m  TranslationStandardAxis=+Z  TranslationCartesianOffset=[0 0 0]  TranslationCartesianOffsetUnits=m  TranslationROffset=0  TranslationROffsetUnits=m  TranslationZOffset=0  TranslationZOffsetUnits=m  TranslationThetaOffset=0  TranslationThetaOffsetUnits=deg  RotationMethod=None  RotationAngleUnits=deg  RotationStandardAxis=+X  RotationAngle=90  RotationArbitraryAxis=[0 0 1]  FollAlignAxisA=+X  BaseAlignAxisA=+Y  FollAlignAxisB=+Y  BaseAlignAxisB=+Z  RotationSequenceAxes=FollowerAxes  RotationSequence=XYX  RotationSequenceAngles=[0 0 0]  RotationSequenceAnglesUnits=deg  RotationMatrix=[1 0 0; 0 1 0; 0 0 1]  Quaternion=[1 0 0 0]
  Earth : sm_lib/Body Elements/Brick Solid  GraphicAmbientColor=[0.15 0.15 0.15 1.0]  BasedOnType=Density  BrickDimensions=[E E P]  BrickDimensionsUnits=m  CenterOfMass=[0 0 0]  CenterOfMassUnits=m  GraphicDiffuseColor=rgbE  Density=rhoE  DensityUnits=kg/m^3  DoExposeReferenceFrame=on  GraphicEmissiveColor=[0.0 0.0 0.0 1.0]  ExportEntireGeometry=on  SerializedFrames=<Frames/>  MarkerShape=Sphere  MarkerSize=10  GraphicType=FromGeometry  InertiaType=CalculateFromGeometry  Mass=1  MassUnits=kg  MomentsOfInertia=[1 1 1]  MomentsOfInertiaUnits=kg*m^2  GraphicOpacity=opE  ProductsOfInertia=[0 0 0]  ProductsOfInertiaUnits=kg*m^2  GraphicShininess=75  GraphicSpecularColor=[0.5 0.5 0.5 1.0]  GraphicVisPropType=SimpleVisualProperties
  Launch Insignia : sm_lib/Body Elements/Extruded Solid  GraphicAmbientColor=[0.15 0.15 0.15 1.0]  BasedOnType=Density  CenterOfMass=[0 0 0]  CenterOfMassUnits=m  GraphicDiffuseColor=[1.0 0.2 0.2]  ExportConvexHullGeometry=off  ExtrusionCrossSection=[0.15 0.15; -0.15 0.15; -0.15 0.75; -0.6 0.75; -0.6 -0.75; -0.15 -0.75; -0.15 -0.15; 0.15 -0.15; 0.15 -0.75; 0.6 -0.75; 0.6 0.75; 0.15 0.75]*0.5  ExtrusionCrossSectionUnits=m  Density=1  DensityUnits=kg/m^3  DoExposeReferenceFrame=on  GraphicEmissiveColor=[0.0 0.0 0.0 1.0]  ExportEntireGeometry=off  ExtrusionLength=0.002  ExtrusionLengthUnits=m  ExtrusionType=General  SerializedFrames=<Frames/>  MarkerShape=Sphere  MarkerSize=10  GraphicType=FromGeometry  InertiaType=CalculateFromGeometry  Mass=1  MassUnits=kg  MomentsOfInertia=[1 1 1]  MomentsOfInertiaUnits=kg*m^2  PolygonNumSides=3  GraphicOpacity=1.0  PolygonOuterRadius=1  PolygonOuterRadiusUnits=m  ProductsOfInertia=[0 0 0]  ProductsOfInertiaUnits=kg*m^2  GraphicShininess=75  GraphicSpecularColor=[0.5 0.5 0.5 1.0]  GraphicVisPropType=SimpleVisualProperties
  Launch Ring : sm_lib/Body Elements/Revolved Solid  GraphicAmbientColor=[0.15 0.15 0.15 1.0]  BasedOnType=Density  CenterOfMass=[0 0 0]  CenterOfMassUnits=m  GraphicDiffuseColor=[0.0 0.2 0.8]  ExportConvexHullGeometry=off  Density=1000  DensityUnits=kg/m^3  DoExposeReferenceFrame=on  GraphicEmissiveColor=[0.0 0.0 0.0 1.0]  ExportEntireGeometry=off  SerializedFrames=<Frames/>  MarkerShape=Sphere  MarkerSize=10  GraphicType=FromGeometry  InertiaType=CalculateFromGeometry  Mass=1  MassUnits=kg  MomentsOfInertia=[1 1 1]  MomentsOfInertiaUnits=kg*m^2  GraphicOpacity=1.0  ProductsOfInertia=[0 0 0]  ProductsOfInertiaUnits=kg*m^2  RevolutionCrossSection=[0.5 0.001; 0.5 -0.001; 0.75 -0.001; 0.75 0.001]  RevolutionCrossSectionUnits=m  RevolutionAngle=180  RevolutionAngleUnits=deg  RevolutionExtent=Full  GraphicShininess=75  GraphicSpecularColor=[0.5 0.5 0.5 1.0]  GraphicVisPropType=SimpleVisualProperties
  Transform Launch : sm_lib/Frames and Transforms/Rigid Transform  TranslationMethod=StandardAxis  TranslationStandardOffset=P/2+Z-0.3  TranslationStandardOffsetUnits=m  TranslationStandardAxis=+Z  TranslationCartesianOffset=P/2+Z+0.01  TranslationCartesianOffsetUnits=m  TranslationROffset=0  TranslationROffsetUnits=m  TranslationZOffset=0  TranslationZOffsetUnits=m  TranslationThetaOffset=0  TranslationThetaOffsetUnits=deg  RotationMethod=None  RotationAngleUnits=deg  RotationStandardAxis=+Z  RotationAngle=0.0  RotationArbitraryAxis=[0 0 1]  FollAlignAxisA=+X  BaseAlignAxisA=+Y  FollAlignAxisB=+Y  BaseAlignAxisB=+Z  RotationSequenceAxes=FollowerAxes  RotationSequence=XYX  RotationSequenceAngles=[0 0 0]  RotationSequenceAnglesUnits=deg  RotationMatrix=[1 0 0; 0 1 0; 0 0 1]  Quaternion=[1 0 0 0]
  Ground : PMIOPort  Side=Right
  Contact : PMIOPort  Port=2  Side=Left
  connections:
  Earth/RConn1 -- Displacement/LConn1
  Contact/RConn1 -- Earth/LConn1
  Ground/RConn1 -- Transform Launch/LConn1 -- Displacement/RConn1
  Launch Ring/RConn1 -- Launch Insignia/RConn1 -- Transform Launch/RConn1

== system Stinger/PLANT MODEL/ENVIRONMENT/Sky ==
  Aft Sky : sm_lib/Body Elements/Brick Solid  GraphicAmbientColor=[0.15 0.15 0.15 1.0]  BasedOnType=Density  BrickDimensions=[E E P]  BrickDimensionsUnits=m  CenterOfMass=[0 0 0]  CenterOfMassUnits=m  GraphicDiffuseColor=rgbS  Density=rhoS  DensityUnits=kg/m^3  DoExposeReferenceFrame=on  GraphicEmissiveColor=[0.0 0.0 0.0 1.0]  ExportEntireGeometry=off  SerializedFrames=<Frames/>  MarkerShape=Sphere  MarkerSize=10  GraphicType=FromGeometry  InertiaType=CalculateFromGeometry  Mass=1  MassUnits=kg  MomentsOfInertia=[1 1 1]  MomentsOfInertiaUnits=kg*m^2  GraphicOpacity=opS  ProductsOfInertia=[0 0 0]  ProductsOfInertiaUnits=kg*m^2  GraphicShininess=75  GraphicSpecularColor=[0.5 0.5 0.5 1.0]  GraphicVisPropType=SimpleVisualProperties
  Displacement1 : sm_lib/Frames and Transforms/Rigid Transform  TranslationMethod=Cartesian  TranslationStandardOffset=E/2  TranslationStandardOffsetUnits=m  TranslationStandardAxis=+Z  TranslationCartesianOffset=[0 -E/2+Z+P E/2+P/2]  TranslationCartesianOffsetUnits=m  TranslationROffset=0  TranslationROffsetUnits=m  TranslationZOffset=0  TranslationZOffsetUnits=m  TranslationThetaOffset=0  TranslationThetaOffsetUnits=deg  RotationMethod=StandardAxis  RotationAngleUnits=deg  RotationStandardAxis=-X  RotationAngle=90  RotationArbitraryAxis=[0 0 1]  FollAlignAxisA=+X  BaseAlignAxisA=+Y  FollAlignAxisB=+Y  BaseAlignAxisB=+Z  RotationSequenceAxes=FollowerAxes  RotationSequence=XYX  RotationSequenceAngles=[0 0 0]  RotationSequenceAnglesUnits=deg  RotationMatrix=[1 0 0; 0 1 0; 0 0 1]  Quaternion=[1 0 0 0]
  Displacement6 : sm_lib/Frames and Transforms/Rigid Transform  TranslationMethod=Cartesian  TranslationStandardOffset=E/2  TranslationStandardOffsetUnits=m  TranslationStandardAxis=+Z  TranslationCartesianOffset=[E/2-Z-P 0 E/2+P/2]  TranslationCartesianOffsetUnits=m  TranslationROffset=0  TranslationROffsetUnits=m  TranslationZOffset=0  TranslationZOffsetUnits=m  TranslationThetaOffset=0  TranslationThetaOffsetUnits=deg  RotationMethod=StandardAxis  RotationAngleUnits=deg  RotationStandardAxis=-Y  RotationAngle=90  RotationArbitraryAxis=[0 0 1]  FollAlignAxisA=+X  BaseAlignAxisA=+Y  FollAlignAxisB=+Y  BaseAlignAxisB=+Z  RotationSequenceAxes=FollowerAxes  RotationSequence=XYX  RotationSequenceAngles=[0 0 0]  RotationSequenceAnglesUnits=deg  RotationMatrix=[1 0 0; 0 1 0; 0 0 1]  Quaternion=[1 0 0 0]
  Left Sky : sm_lib/Body Elements/Brick Solid  GraphicAmbientColor=[0.15 0.15 0.15 1.0]  BasedOnType=Density  BrickDimensions=[E E P]  BrickDimensionsUnits=m  CenterOfMass=[0 0 0]  CenterOfMassUnits=m  GraphicDiffuseColor=rgbS  Density=rhoS  DensityUnits=kg/m^3  DoExposeReferenceFrame=on  GraphicEmissiveColor=[0.0 0.0 0.0 1.0]  ExportEntireGeometry=off  SerializedFrames=<Frames/>  MarkerShape=Sphere  MarkerSize=10  GraphicType=FromGeometry  InertiaType=CalculateFromGeometry  Mass=1  MassUnits=kg  MomentsOfInertia=[1 1 1]  MomentsOfInertiaUnits=kg*m^2  GraphicOpacity=opS  ProductsOfInertia=[0 0 0]  ProductsOfInertiaUnits=kg*m^2  GraphicShininess=75  GraphicSpecularColor=[0.5 0.5 0.5 1.0]  GraphicVisPropType=SimpleVisualProperties
  Sky : PMIOPort  Side=Right
  connections:
  Displacement6/LConn1 -- Left Sky/RConn1
  Displacement1/LConn1 -- Aft Sky/RConn1
  Sky/RConn1 -- Displacement1/RConn1 -- Displacement6/RConn1

== system Stinger/PLANT MODEL/ENVIRONMENT/Tree ==
  File Solid : sm_lib/Body Elements/File Solid  ExtGeomFileName=UAV_VirtualPrototyping\STL files\Tree.stl  UnitType=Custom  ExtGeomFileUnits=mm  StepReaderType=HEX  ExportConvexHullGeometry=off  InertiaType=PointMass  Mass=1  MassUnits=kg  CenterOfMass=[0 0 0]  CenterOfMassUnits=m  MomentsOfInertia=[1 1 1]  MomentsOfInertiaUnits=kg*m^2  ProductsOfInertia=[0 0 0]  ProductsOfInertiaUnits=kg*m^2  BasedOnType=DensityFromFile  Density=1000  DensityUnits=kg/m^3  DoExposeReferenceFrame=on  SerializedFrames=<Frames/>  GraphicType=FromGeometry  MarkerShape=Sphere  MarkerSize=10  GraphicVisPropType=SimpleVisualProperties  GraphicDiffuseColor=[0.0 0.6 0.0]  GraphicSpecularColor=[0.5 0.5 0.5 1.0]  GraphicAmbientColor=[0.15 0.15 0.15 1.0]  GraphicEmissiveColor=[0.0 0.0 0.0 1.0]  GraphicShininess=75  GraphicOpacity=1.0
  Rigid Transform : sm_lib/Frames and Transforms/Rigid Transform  TranslationMethod=Cartesian  TranslationStandardOffset=0  TranslationStandardOffsetUnits=m  TranslationStandardAxis=+Z  TranslationCartesianOffset=[E/2-3 -2 0.2]  TranslationCartesianOffsetUnits=m  TranslationROffset=0  TranslationROffsetUnits=m  TranslationZOffset=0  TranslationZOffsetUnits=m  TranslationThetaOffset=0  TranslationThetaOffsetUnits=deg  RotationMethod=None  RotationAngleUnits=deg  RotationStandardAxis=+Z  RotationAngle=0.0  RotationArbitraryAxis=[0 0 1]  FollAlignAxisA=+X  BaseAlignAxisA=+Y  FollAlignAxisB=+Y  BaseAlignAxisB=+Z  RotationSequenceAxes=FollowerAxes  RotationSequence=XYX  RotationSequenceAngles=[0 0 0]  RotationSequenceAnglesUnits=deg  RotationMatrix=[1 0 0; 0 1 0; 0 0 1]  Quaternion=[1 0 0 0]
  Buildings : PMIOPort  Side=Right
  connections:
  Rigid Transform/RConn1 -- Buildings/RConn1
  File Solid/RConn1 -- Rigid Transform/LConn1

== system Stinger/PLANT MODEL/SENSORS/Quaternion to Rotation Angles ==
  q : Inport  Unit=1
  Angle Calculation : sharedtransformsys/Non-Singular  rot=ZYX  aMode=aMode
  Quaternion Normalize : sharedutil/Quaternion Normalize  aMode=aMode
  fcn1 : Fcn  Expr=2*(u[2]*u[3] + u[1]*u[4])
  fcn2 : Fcn  Expr=u[1]*u[1] + u[2]*u[2] - u[3]*u[3] - u[4]*u[4]
  fcn3 : Fcn  Expr=-2*(u[2]*u[4] - u[1]*u[3])
  fcn4 : Fcn  Expr=2*(u[3]*u[4] + u[1]*u[2])
  fcn5 : Fcn  Expr=u[1]*u[1] - u[2]*u[2] - u[3]*u[3] + u[4]*u[4]
  R1,R2,R3 : Outport  Unit=rad  VectorParamsAs1DForOutWhenUnconnected=off
  wires:
  fcn3/1 -> Angle Calculation/4
  fcn2/1 -> Angle Calculation/3
  Quaternion Normalize/1 -> fcn3/1, fcn4/1, fcn5/1, fcn2/1, fcn1/1
  q/1 -> Quaternion Normalize/1, Angle Calculation/1
  Angle Calculation/1 -> R1,R2,R3/1
  fcn5/1 -> Angle Calculation/6
  fcn1/1 -> Angle Calculation/2
  fcn4/1 -> Angle Calculation/5

== system Stinger/PLANT MODEL/ELECTRIC SYSTEM/Motor 1/RPM to Resistive Torque and Thrust1 ==
  Angular Speed : Inport
  Constant : Constant  Value=0
  From : From  Commented=on  GotoTag=Velocity  TagVisibility=global
  Gain : Gain  Gain=-1
  Thrust & Torque Based on Propeller Rotational and Translational Velocity : MATLAB Function  TreatAsAtomicUnit=on
  Thrust : Outport
  Resistive Torque : Outport  Port=2
  wires:
  Gain/1 -> Resistive Torque/1
  Constant/1 -> Thrust & Torque Based on Propeller Rotational and Translational Velocity/1(Velocity)
  Thrust & Torque Based on Propeller Rotational and Translational Velocity/2(Torque) -> Gain/1
  Angular Speed/1 -> Thrust & Torque Based on Propeller Rotational and Translational Velocity/2(RPM)  "Speed"
  Thrust & Torque Based on Propeller Rotational and Translational Velocity/1(Thrust) -> Thrust/1

== system Stinger/PLANT MODEL/ELECTRIC SYSTEM/Motor 1/Signals ==
  Mux : Mux  Inputs=2
      settings: DisplayOption=signals
  Spd : Outport  VectorParamsAs1DForOutWhenUnconnected=off
  ia : Outport  Port=2  VectorParamsAs1DForOutWhenUnconnected=off
  Trq : Outport  Port=3  VectorParamsAs1DForOutWhenUnconnected=off
  V : Outport  Port=4  VectorParamsAs1DForOutWhenUnconnected=off
  wires:
  [Trq1] -> Trq/1  "Motor torque [N*m]"
  [AngularSpeed1] -> Mux/2  "actual speed"
  Mux/1 -> Spd/1  "Requested and measured velocity [rpm]"
  [ReqSpeedMotor1] -> Mux/1  "req speed"
  [ia] -> ia/1  "Armature current [A]"
  [voltage] -> V/1  "Motor Voltage (V)"

== system Stinger/PLANT MODEL/ELECTRIC SYSTEM/Motor 2/RPM to Resistive Torque and Thrust ==
  Angular Speed : Inport
  Constant : Constant  Value=0
  From : From  Commented=on  GotoTag=Velocity  TagVisibility=global
  Gain : Gain  Gain=-1
  Thrust & Torque Based on Propeller Rotational and Translational Velocity : MATLAB Function  TreatAsAtomicUnit=on
  Thrust : Outport
  Resistive Torque : Outport  Port=2
  wires:
  Gain/1 -> Resistive Torque/1
  Constant/1 -> Thrust & Torque Based on Propeller Rotational and Translational Velocity/1(Velocity)
  Thrust & Torque Based on Propeller Rotational and Translational Velocity/2(Torque) -> Gain/1
  Angular Speed/1 -> Thrust & Torque Based on Propeller Rotational and Translational Velocity/2(RPM)  "Speed"
  Thrust & Torque Based on Propeller Rotational and Translational Velocity/1(Thrust) -> Thrust/1

== system Stinger/PLANT MODEL/ELECTRIC SYSTEM/Motor 3/RPM to Resistive Torque and Thrust ==
  Angular Speed : Inport
  Constant : Constant  Value=0
  From : From  Commented=on  GotoTag=Velocity  TagVisibility=global
  Gain : Gain  Gain=-1
  Thrust & Torque Based on Propeller Rotational and Translational Velocity : MATLAB Function  TreatAsAtomicUnit=on
  Thrust : Outport
  Resistive Torque : Outport  Port=2
  wires:
  Gain/1 -> Resistive Torque/1
  Constant/1 -> Thrust & Torque Based on Propeller Rotational and Translational Velocity/1(Velocity)
  Thrust & Torque Based on Propeller Rotational and Translational Velocity/2(Torque) -> Gain/1
  Angular Speed/1 -> Thrust & Torque Based on Propeller Rotational and Translational Velocity/2(RPM)  "Speed"
  Thrust & Torque Based on Propeller Rotational and Translational Velocity/1(Thrust) -> Thrust/1

== system Stinger/PLANT MODEL/ELECTRIC SYSTEM/Motor 4/RPM to Resistive Torque and Thrust ==
  Angular Speed : Inport
  Constant : Constant  Value=0
  From : From  Commented=on  GotoTag=Velocity  TagVisibility=global
  Gain : Gain  Gain=-1
  Thrust & Torque Based on Propeller Rotational and Translational Velocity : MATLAB Function  TreatAsAtomicUnit=on
  Thrust : Outport
  Resistive Torque : Outport  Port=2
  wires:
  Gain/1 -> Resistive Torque/1
  Constant/1 -> Thrust & Torque Based on Propeller Rotational and Translational Velocity/1(Velocity)
  Thrust & Torque Based on Propeller Rotational and Translational Velocity/2(Torque) -> Gain/1
  Angular Speed/1 -> Thrust & Torque Based on Propeller Rotational and Translational Velocity/2(RPM)  "Speed"
  Thrust & Torque Based on Propeller Rotational and Translational Velocity/1(Thrust) -> Thrust/1

== system Stinger/PLANT MODEL/ELECTRIC SYSTEM/Motor 5/RPM to Resistive Torque and Thrust ==
  Angular Speed : Inport
  Constant : Constant  Value=0
  From : From  Commented=on  GotoTag=Velocity  TagVisibility=global
  Gain : Gain  Gain=-1
  Thrust & Torque Based on Propeller Rotational and Translational Velocity : MATLAB Function  TreatAsAtomicUnit=on
  Thrust : Outport
  Resistive Torque : Outport  Port=2
  wires:
  Gain/1 -> Resistive Torque/1
  Constant/1 -> Thrust & Torque Based on Propeller Rotational and Translational Velocity/1(Velocity)
  Thrust & Torque Based on Propeller Rotational and Translational Velocity/2(Torque) -> Gain/1
  Angular Speed/1 -> Thrust & Torque Based on Propeller Rotational and Translational Velocity/2(RPM)  "Speed"
  Thrust & Torque Based on Propeller Rotational and Translational Velocity/1(Thrust) -> Thrust/1

== system Stinger/PLANT MODEL/ELECTRIC SYSTEM/Motor 6/RPM to Resistive Torque and Thrust ==
  Angular Speed : Inport
  Constant : Constant  Value=0
  From : From  Commented=on  GotoTag=Velocity  TagVisibility=global
  Gain : Gain  Gain=-1
  Thrust & Torque Based on Propeller Rotational and Translational Velocity : MATLAB Function  TreatAsAtomicUnit=on
  Thrust : Outport
  Resistive Torque : Outport  Port=2
  wires:
  Gain/1 -> Resistive Torque/1
  Constant/1 -> Thrust & Torque Based on Propeller Rotational and Translational Velocity/1(Velocity)
  Thrust & Torque Based on Propeller Rotational and Translational Velocity/2(Torque) -> Gain/1
  Angular Speed/1 -> Thrust & Torque Based on Propeller Rotational and Translational Velocity/2(RPM)  "Speed"
  Thrust & Torque Based on Propeller Rotational and Translational Velocity/1(Thrust) -> Thrust/1
